simulink model "highpass_test"  (R2016b)
settings: Solver=VariableStepAuto  StartTime=0.0  StopTime=10  RelTol=1e-3
undefined symbols (not defined in the file or in its folder): T
settings Model: Creator=michael  LastModifiedBy=michael

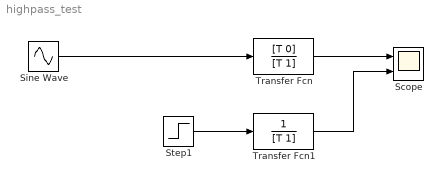
== system highpass_test ==
  Scope : Scope  NumInputPorts=2
  Sine Wave : Sin  Frequency=2*pi*5  SampleTime=0
  Step1 : Step  SampleTime=0
  Transfer Fcn : TransferFcn  Numerator=[T 0]  Denominator=[T 1]
  Transfer Fcn1 : TransferFcn  Denominator=[T 1]
  wires:
  Sine Wave/1 -> Transfer Fcn/1
  Transfer Fcn/1 -> Scope/1
  Step1/1 -> Transfer Fcn1/1
  Transfer Fcn1/1 -> Scope/2
